simulink model "parallel_fp_fra"  (R2023a)
settings: Solver=VariableStepAuto  StartTime=0.0  StopTime=10.0  RelTol=1e-3
undefined symbols (not defined in the file): dqi, fd, invMd, K, KD, KF, KI, KP, Md, qi, robot, xd, xr
settings Model: Creator=franc  LastModifiedBy=franc

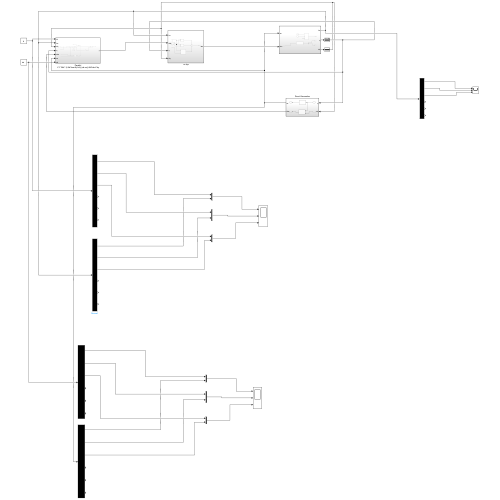
[thumbnail: Simulink's stored preview of the top-level diagram]
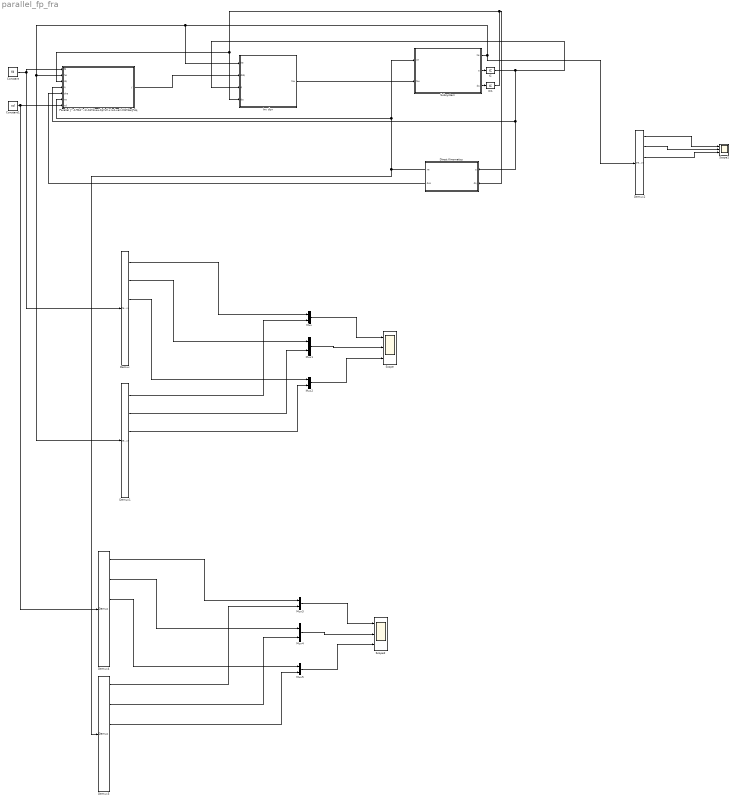
== system parallel_fp_fra ==
  Constant : Constant  Value=fd
  Constant1 : Constant  Value=xd
  Demux{,1..4} (5 alike) : Demux  Outputs=6
  Direct Kinematics : Subsystem
  IC : InitialCondition  Value=[0 0 0]
  IC1 : InitialCondition  Value=[0 0 0]
  Inv dyn : Subsystem
  Mux{,1..5} (6 alike) : Mux  Inputs=2
  Parallel J^-1*Md^-1(-Kd*dxe+Kp*xf(+(xd-xe))-Md*derJ*dq : Subsystem
  Scope : Scope  NumInputPorts=3
  Scope1 : Scope  NumInputPorts=3
  Scope2 : Scope  NumInputPorts=3
  Subsystem : Subsystem
  wires:
  Demux1/3 -> Mux2/2
  Mux1/1 -> Scope/2
  Demux2/1 -> Scope1/1
  Demux1/2 -> Mux1/2
  Mux/1 -> Scope/1
  Demux/3 -> Mux2/1
  Demux/2 -> Mux1/1
  Demux2/2 -> Scope1/2
  Demux1/1 -> Mux/2
  Constant/1 -> Parallel J^-1*Md^-1(-Kd*dxe+Kp*xf(+(xd-xe))-Md*derJ*dq/1(fd), Demux/1
  Parallel J^-1*Md^-1(-Kd*dxe+Kp*xf(+(xd-xe))-Md*derJ*dq/1(y) -> Inv dyn/2(ddq)
  Direct Kinematics/2(dxe) -> Parallel J^-1*Md^-1(-Kd*dxe+Kp*xf(+(xd-xe))-Md*derJ*dq/5(dxe)
  Mux2/1 -> Scope/3
  Subsystem/1(he) -> Demux2/1, Inv dyn/1(he), Demux1/1, Parallel J^-1*Md^-1(-Kd*dxe+Kp*xf(+(xd-xe))-Md*derJ*dq/2(he)
  IC/1 -> Parallel J^-1*Md^-1(-Kd*dxe+Kp*xf(+(xd-xe))-Md*derJ*dq/4(q), Direct Kinematics/1(q), Inv dyn/3(q)
  Subsystem/3(dq) -> IC1/1
  Inv dyn/1(tau) -> Subsystem/2(tau)
  Demux2/3 -> Scope1/3
  Demux/1 -> Mux/1
  Direct Kinematics/1(xe) -> Demux3/1, Subsystem/1(xe), Parallel J^-1*Md^-1(-Kd*dxe+Kp*xf(+(xd-xe))-Md*derJ*dq/6(xe)
  Subsystem/2(q) -> IC/1
  IC1/1 -> Parallel J^-1*Md^-1(-Kd*dxe+Kp*xf(+(xd-xe))-Md*derJ*dq/3(dq), Inv dyn/4(dq), Direct Kinematics/2(dq)
  Constant1/1 -> Demux4/1, Parallel J^-1*Md^-1(-Kd*dxe+Kp*xf(+(xd-xe))-Md*derJ*dq/7(xd)
  Mux5/1 -> Scope2/3
  Mux4/1 -> Scope2/2
  Mux3/1 -> Scope2/1
  Demux4/1 -> Mux3/1
  Demux4/2 -> Mux4/1
  Demux4/3 -> Mux5/1
  Demux3/1 -> Mux3/2
  Demux3/2 -> Mux4/2
  Demux3/3 -> Mux5/2

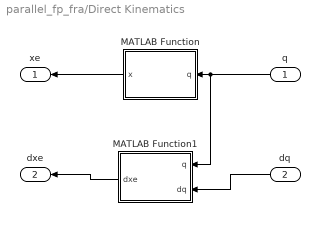
== system parallel_fp_fra/Direct Kinematics ==
  q : Inport
  dq : Inport  Port=2
  MATLAB Function : MATLAB Function  TreatAsAtomicUnit=on
  MATLAB Function1 : MATLAB Function  TreatAsAtomicUnit=on
  xe : Outport
  dxe : Outport  Port=2
  wires:
  dq/1 -> MATLAB Function1/2(dq)
  MATLAB Function1/1(dxe) -> dxe/1
  MATLAB Function/1(x) -> xe/1
  q/1 -> MATLAB Function/1(q), MATLAB Function1/1(q)

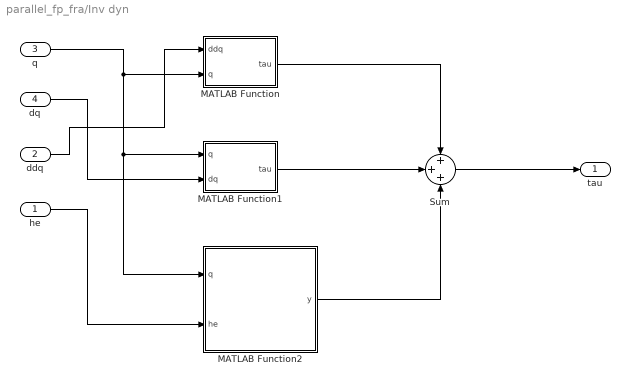
== system parallel_fp_fra/Inv dyn ==
  he : Inport
  ddq : Inport  Port=2
  q : Inport  Port=3
  dq : Inport  Port=4
  MATLAB Function : MATLAB Function  TreatAsAtomicUnit=on
  MATLAB Function1 : MATLAB Function  TreatAsAtomicUnit=on
  MATLAB Function2 : MATLAB Function  TreatAsAtomicUnit=on
  Sum : Sum  Inputs=+++
  tau : Outport
  wires:
  Sum/1 -> tau/1
  MATLAB Function1/1(tau) -> Sum/2
  MATLAB Function/1(tau) -> Sum/1
  MATLAB Function2/1(y) -> Sum/3
  q/1 -> MATLAB Function/2(q), MATLAB Function2/1(q), MATLAB Function1/1(q)
  dq/1 -> MATLAB Function1/2(dq)
  he/1 -> MATLAB Function2/2(he)
  ddq/1 -> MATLAB Function/1(ddq)

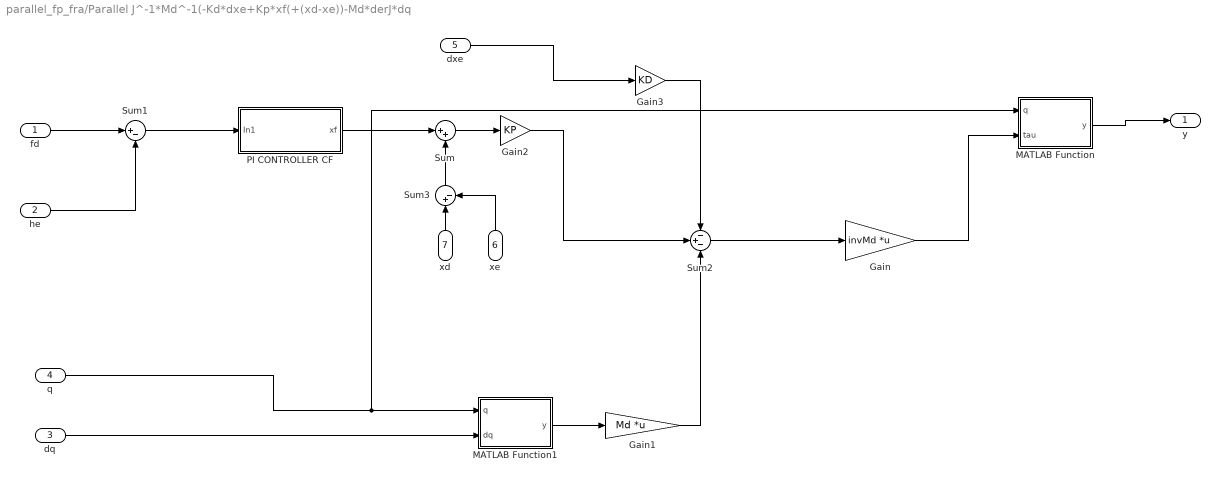
== system parallel_fp_fra/Parallel J^-1*Md^-1(-Kd*dxe+Kp*xf(+(xd-xe))-Md*derJ*dq ==
  fd : Inport
  he : Inport  Port=2
  dq : Inport  Port=3
  q : Inport  Port=4
  dxe : Inport  Port=5
  xe : Inport  Port=6
  xd : Inport  Port=7
  Gain : Gain  Gain=invMd  Multiplication=Matrix(K*u)
  Gain1 : Gain  Gain=Md  Multiplication=Matrix(K*u)
  Gain2 : Gain  Gain=KP
  Gain3 : Gain  Gain=KD
  MATLAB Function : MATLAB Function  TreatAsAtomicUnit=on
  MATLAB Function1 : MATLAB Function  TreatAsAtomicUnit=on
  PI CONTROLLER CF : Subsystem
  Sum : Sum  Inputs=|++
  Sum1 : Sum  Inputs=|+-
  Sum2 : Sum  Inputs=-+-
  Sum3 : Sum  Inputs=|+-
  y : Outport
  wires:
  fd/1 -> Sum1/1
  Sum1/1 -> PI CONTROLLER CF/1(In1)
  he/1 -> Sum1/2
  MATLAB Function/1(y) -> y/1
  Gain/1 -> MATLAB Function/2(tau)
  Sum2/1 -> Gain/1
  MATLAB Function1/1(y) -> Gain1/1
  Gain1/1 -> Sum2/3
  dq/1 -> MATLAB Function1/2(dq)
  q/1 -> MATLAB Function/1(q), MATLAB Function1/1(q)
  Gain2/1 -> Sum2/2
  dxe/1 -> Gain3/1
  Gain3/1 -> Sum2/1
  Sum/1 -> Gain2/1
  PI CONTROLLER CF/1(xf) -> Sum/1
  xe/1 -> Sum3/2
  xd/1 -> Sum3/1
  Sum3/1 -> Sum/2

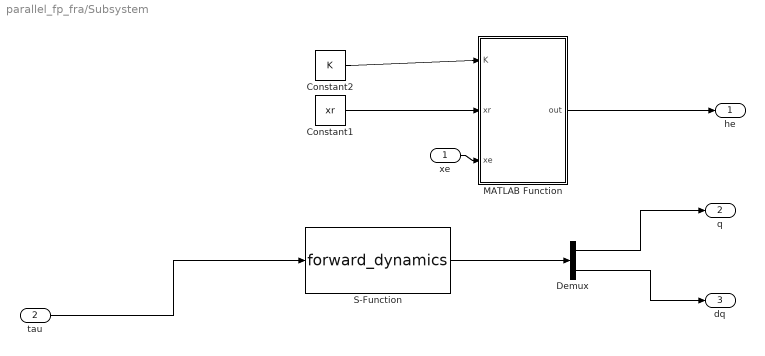
== system parallel_fp_fra/Subsystem ==
  xe : Inport
  tau : Inport  Port=2
  Constant1 : Constant  Value=xr
  Constant2 : Constant  Value=K
  Demux : Demux  Outputs=2
  MATLAB Function : MATLAB Function  TreatAsAtomicUnit=on
  S-Function : S-Function  FunctionName=forward_dynamics  Parameters=robot,qi,dqi  SFunctionDeploymentMode=off  EnableBusSupport=off
  he : Outport
  q : Outport  Port=2
  dq : Outport  Port=3
  wires:
  S-Function/1 -> Demux/1
  Constant2/1 -> MATLAB Function/1(K)
  Demux/1 -> q/1
  Constant1/1 -> MATLAB Function/2(xr)
  xe/1 -> MATLAB Function/3(xe)
  MATLAB Function/1(out) -> he/1
  tau/1 -> S-Function/1
  Demux/2 -> dq/1

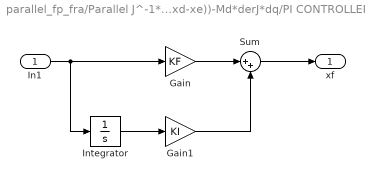
== system parallel_fp_fra/Parallel J^-1*Md^-1(-Kd*dxe+Kp*xf(+(xd-xe))-Md*derJ*dq/PI CONTROLLER CF ==
  In1 : Inport
  Gain : Gain  Gain=KF
  Gain1 : Gain  Gain=KI
  Integrator : Integrator
  Sum : Sum  Inputs=|++
  xf : Outport
  wires:
  Integrator/1 -> Gain1/1
  In1/1 -> Gain/1, Integrator/1
  Gain/1 -> Sum/1
  Gain1/1 -> Sum/2
  Sum/1 -> xf/1

== matlab function parallel_fp_fra/Parallel J^-1*Md^-1(-Kd*dxe+Kp*xf(+(xd-xe))-Md*derJ*dq/MATLAB Function ==
  data: q input; y output; tau input
function y = inv_J(q,tau)

y = get_Ja_inverse_as_9(q(1),q(2),q(3))*tau;

== matlab function parallel_fp_fra/Inv dyn/MATLAB Function ==
  data: ddq input; tau output; q input
function tau = B(ddq, q)

tau = get_B_as_7(q(1),q(3))*ddq;

== matlab function parallel_fp_fra/Inv dyn/MATLAB Function1 ==
  data: q input; tau output; dq input
function tau = n(q, dq)

tau = get_n_as_7(q(1),q(3),dq(1),dq(3));

== matlab function parallel_fp_fra/Inv dyn/MATLAB Function2 ==
  data: q input; y output; he input
function y = operational_he(q,he)

y = get_Ja_as_9(q(1),q(2),q(3))'*he;

== matlab function parallel_fp_fra/Subsystem/MATLAB Function ==
  data: K input; out output; xr input; xe input
function out = environment(K,xr, xe)
%consider the interaction only in z direction
if xe(3) > xr(3)
    out = K*(xe-xr);
else 
    out = zeros(6,1);
end

== matlab function parallel_fp_fra/Direct Kinematics/MATLAB Function ==
  data: q input; x output
function x = getK(q)

x = new_getK(q);

== matlab function parallel_fp_fra/Direct Kinematics/MATLAB Function1 ==
  data: q input; dxe output; dq input
function dxe = Ja(q,dq)

dxe = get_Ja_as_9(q(1),q(2),q(3))*dq;

== matlab function parallel_fp_fra/Parallel J^-1*Md^-1(-Kd*dxe+Kp*xf(+(xd-xe))-Md*derJ*dq/MATLAB Function1 ==
  data: q input; y output; dq input
function y = der_J(q,dq)

y = get_derivative_Ja_as_9(q(1),q(2),q(3),dq(1),dq(2),dq(3))*dq;
